simulink model "pendulum"  (R2021b)
settings: Solver=VariableStepAuto  StartTime=0.0  StopTime=10.0  RelTol=1e-3
settings Model: Creator=CC319  LastModifiedBy=CC319

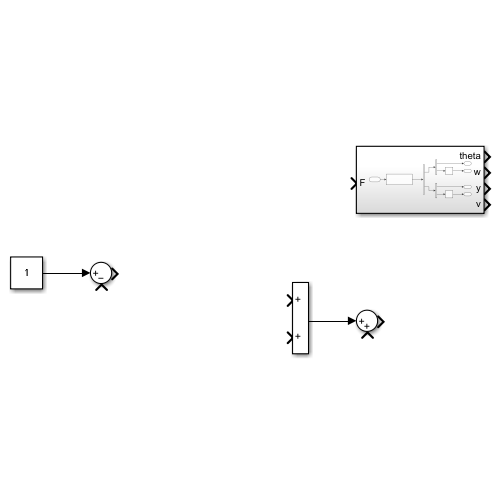
[thumbnail: Simulink's stored preview of the top-level diagram]
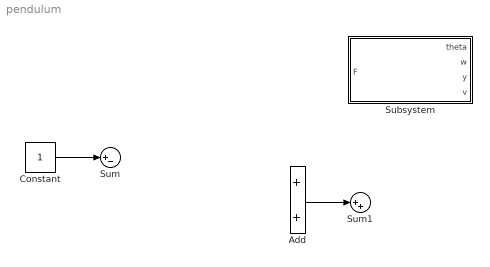
== system pendulum ==
  Add : Sum
  Constant : Constant
  Subsystem : Subsystem
  Sum : Sum  Inputs=|+-
  Sum1 : Sum  Inputs=|++
  wires:
  Constant/1 -> Sum/1
  Add/1 -> Sum1/1

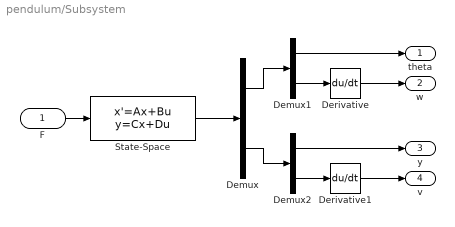
== system pendulum/Subsystem ==
  F : Inport
  Demux : Demux  Outputs=2
  Demux1 : Demux  Outputs=2
  Demux2 : Demux  Outputs=2
  Derivative : Derivative
  Derivative1 : Derivative
  State-Space : StateSpace  A=[0 1 0 0;14.8531 0 0 0;0 0 0 1;-7.0335 0 0 0]  B=[0;-0.1407;0;0.0160]  C=[1 0 0 0;0 0 1 0]  D=[0;0]  InitialCondition=0
  theta : Outport
  w : Outport  Port=2
  y : Outport  Port=3
  v : Outport  Port=4
  wires:
  State-Space/1 -> Demux/1
  Demux/2 -> Demux2/1
  Demux/1 -> Demux1/1
  F/1 -> State-Space/1
  Demux1/2 -> Derivative/1
  Demux2/2 -> Derivative1/1
  Demux1/1 -> theta/1
  Derivative/1 -> w/1
  Demux2/1 -> y/1
  Derivative1/1 -> v/1
